simulink library "constantUniformFlow_ul"  (R2018b)
settings: Solver=VariableStepAuto  StartTime=0.0  StopTime=10.0  RelTol=1e-3
undefined symbols (not defined in the file or in its folder): env, initializeBussesFromBlock
settings Model: Creator=mcobb  LastModifiedBy=mcobb

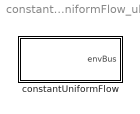
== system constantUniformFlow_ul ==
  constantUniformFlow : Subsystem  LoadFcn=initializeBussesFromBlock(gcb)  InitFcn=initializeBussesFromBlock(gcb)  StartFcn=initializeBussesFromBlock(gcb)  VariantControl=VSS_environment_constantUniformFlow
      settings: PostSaveFcn=initializeBussesFromBlock(gcb)

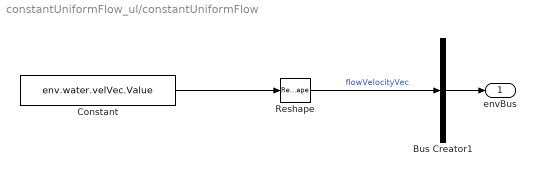
== system constantUniformFlow_ul/constantUniformFlow ==
  Bus Creator1 : BusCreator  Inputs=1  OutDataTypeStr=Bus:envBus
  Constant : Constant  Value=env.water.velVec.Value
  Reshape : Reshape  OutputDimensionality=Column vector (2-D)
  envBus : Outport  OutDataTypeStr=Bus: envBus
  wires:
  Bus Creator1/1 -> envBus/1
  Reshape/1 -> Bus Creator1/1  "flowVelocityVec"
  Constant/1 -> Reshape/1
